simulink model "Electric_Bike"  (R2021a)
settings: Solver=VariableStepAuto  StartTime=0.0  StopTime=5  RelTol=1e-3
values from neighbouring files (symbols this model uses):
  A = [-Rm/Lm -Kb/Lm; Kt/Jeq -Beq/Jeq]    [Electric_Bicycle.m]
  AO = [A-L*C]    [Electric_Bicycle.m]
  B = [1/Lm 0;0 1/(Jeq*Em)]    [Electric_Bicycle.m]
  Beq = Bm+(B/((Em^2)*(Eg^2)))    (= 0.000601487896416)    [Electric_Bicycle.m]
  BO = [B L]    [Electric_Bicycle.m]
  C = [0 1/(Em*Eg)]    [Electric_Bicycle.m]
  CO = eye(2)    [Electric_Bicycle.m]
  DO = zeros(2,3)    [Electric_Bicycle.m]
  Eg = 0.73    [Electric_Bicycle.m]
  Em = 25    [Electric_Bicycle.m]
  Jeq = Jm+(Jb/((Em^2)*(Eg^2)))    (= 0.0135299776694)    [Electric_Bicycle.m]
  Kb = 0.16    [Electric_Bicycle.m]
  kc = place(A,B,[p1 p2])    [Electric_Bicycle.m]
  Kt = 0.16    [Electric_Bicycle.m]
  Lm = 0.003    [Electric_Bicycle.m]
  Rm = 0.85    [Electric_Bicycle.m]
settings Model: Creator=Ferna  LastModifiedBy=Ferna

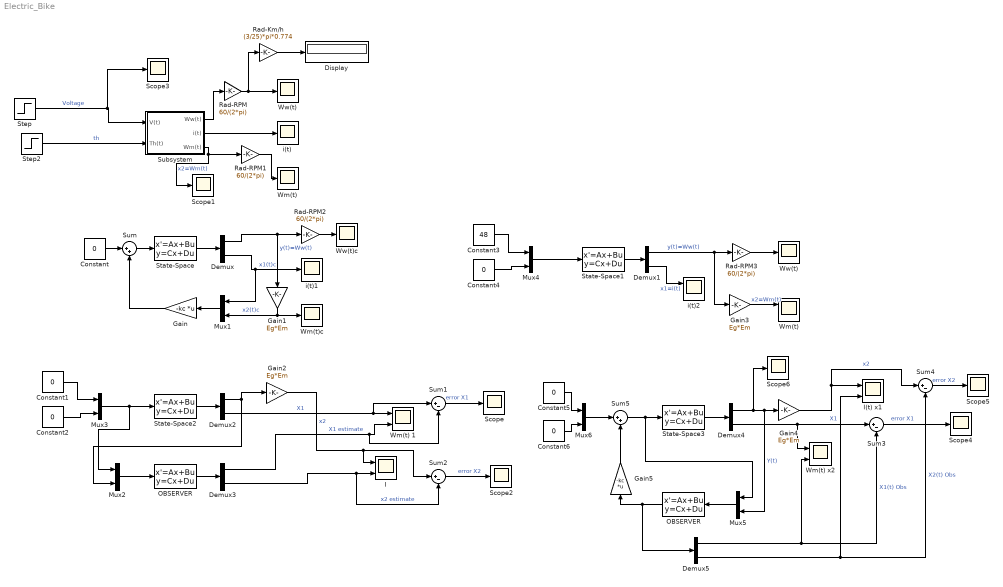
== system Electric_Bike ==
  Constant{,1..2,4..6} (6 alike) : Constant  Value=0
  Constant3 : Constant  Value=48
  Demux{,1..5} (6 alike) : Demux  Outputs=2
  Display : Display
  Gain : Gain  Gain=-kc  Multiplication=Matrix(K*u)
  Gain{1..4} (4 alike) : Gain  Gain=Eg*Em
  Gain5 : Gain  Gain=-kc  Multiplication=Matrix(K*u)
  I : Scope  NumInputPorts=2
  I(t) x1 : Scope  NumInputPorts=2
  Mux{1..6} (6 alike) : Mux  Inputs=2
  OBSERVER : StateSpace  A=AO  B=BO  C=CO  D=DO  InitialCondition=[0 100]
  "OBSERVER " : StateSpace  A=AO  B=BO  C=CO  D=DO  InitialCondition=[0 100]
  Rad-Km/h : Gain  Gain=(3/25)*pi*0.774
  Rad-RPM{,1..3} (4 alike) : Gain  Gain=60/(2*pi)
  Scope{,1..6} (7 alike) : Scope
  State-Space : StateSpace  A=A  B=B  C=[C;1 0]  D=[0 0;0 0]  InitialCondition=[0 100]
  State-Space1 : StateSpace  A=A  B=B  C=[C;1 0]  D=[0 0;0 0]  InitialCondition=[0 0]
  State-Space2 : StateSpace  A=A  B=B  C=[C;1 0]  D=[0 0;0 0]  InitialCondition=[0 100]
  State-Space3 : StateSpace  A=A  B=B  C=[C;1 0]  D=[0 0;0 0]  InitialCondition=[0 100]
  Step : Step  After=12  SampleTime=0
  Step2 : Step  After=69.3  SampleTime=0
  Subsystem : Subsystem
  Sum : Sum  Inputs=|++
  Sum{1..4} (4 alike) : Sum  Inputs=|+-
  Sum5 : Sum  Inputs=|++
  Wm(t) : Scope
  "Wm(t) " : Scope  NumInputPorts=2
  Wm(t) 1 : Scope  NumInputPorts=2
  Wm(t) x2 : Scope  NumInputPorts=2
  Wm(t)c : Scope
  Ww(t) : Scope
  "Ww(t) " : Scope
  Ww(t)c : Scope
  "i(t) " : Scope
  i(t)1 : Scope
  i(t)2 : Scope  NumInputPorts=2
  wires:
  Subsystem/2(i(t)) -> "i(t) "/1
  Subsystem/1(Ww(t)) -> Rad-RPM/1
  Subsystem/3(Wm(t)) -> Scope1/1, Rad-RPM1/1  "x2=Wm(t)"
  Rad-RPM/1 -> Rad-Km/h/1, Ww(t)/1
  Rad-RPM1/1 -> Wm(t)/1
  Rad-Km/h/1 -> Display/1
  Step/1 -> Scope3/1, Subsystem/1(V(t))  "Voltage"
  Step2/1 -> Subsystem/2(Th(t))  "th"
  State-Space/1 -> Demux/1
  Demux/2 -> Mux1/1, i(t)1/1  "x1(t)c"
  Demux/1 -> Rad-RPM2/1, Gain1/1  "y(t)=Ww(t)"
  Rad-RPM2/1 -> Ww(t)c/1
  Mux1/1 -> Gain/1
  Sum/1 -> State-Space/1
  Gain1/1 -> Mux1/2, Wm(t)c/1  "x2(t)c"
  Gain/1 -> Sum/2
  Gain3/1 -> "Wm(t) "/1  "x2=Wm(t)"
  Demux1/1 -> Rad-RPM3/1, Gain3/1  "y(t)=Ww(t)"
  Rad-RPM3/1 -> "Ww(t) "/1
  Demux1/2 -> i(t)2/1  "x1=i(t)"
  State-Space1/1 -> Demux1/1
  Constant/1 -> Sum/1
  Mux2/1 -> OBSERVER/1
  Mux3/1 -> Mux2/1, State-Space2/1
  Constant1/1 -> Mux3/1
  Constant2/1 -> Mux3/2
  Mux4/1 -> State-Space1/1
  Constant3/1 -> Mux4/1
  Constant4/1 -> Mux4/2
  State-Space2/1 -> Demux2/1
  Demux2/1 -> Gain2/1, Mux2/2
  OBSERVER/1 -> Demux3/1
  Demux3/2 -> I/2, Sum2/2  "x2 estimate"
  Demux3/1 -> Sum1/2, Wm(t) 1/2  "X1 estimate"
  Demux2/2 -> Sum1/1, Wm(t) 1/1  "X1"
  Gain2/1 -> I/1, Sum2/1  "x2"
  Sum1/1 -> Scope/1  "error X1"
  Sum2/1 -> Scope2/1  "error X2"
  Sum4/1 -> Scope5/1  "error X2"
  State-Space3/1 -> Demux4/1
  Demux4/2 -> Sum3/1, Wm(t) x2/1  "X1"
  Gain4/1 -> Sum4/1, I(t) x1/1  "x2"
  Mux5/1 -> "OBSERVER "/1
  Constant5/1 -> Mux6/1
  Demux4/1 -> Scope6/1, Mux5/2, Gain4/1  "Y(t)"
  Sum3/1 -> Scope4/1  "error X1"
  Constant6/1 -> Mux6/2
  "OBSERVER "/1 -> Demux5/1, Gain5/1
  Sum5/1 -> Mux5/1, State-Space3/1
  Gain5/1 -> Sum5/2
  Mux6/1 -> Sum5/1
  Demux5/1 -> Wm(t) x2/2, Sum3/2  "X1(t) Obs"
  Demux5/2 -> Sum4/2, I(t) x1/2  "X2(t) Obs"

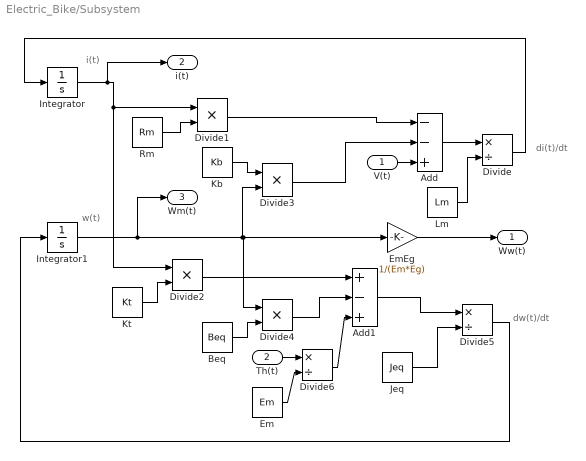
== system Electric_Bike/Subsystem ==
  note: i(t)
  note: w(t)
  note: di(t)/dt
  note: dw(t)/dt
  V(t) : Inport
  Th(t) : Inport  Port=2
  Add : Sum  Inputs=--+
  Add1 : Sum  Inputs=+-+
  Beq : Constant  Value=Beq
  Divide : Product  Inputs=*/
  Divide{1..4} (4 alike) : Product  Inputs=**
  Divide5 : Product  Inputs=*/
  Divide6 : Product  Inputs=*/
  Em : Constant  Value=Em
  EmEg : Gain  Gain=1/(Em*Eg)
  Integrator : Integrator
  Integrator1 : Integrator
  Jeq : Constant  Value=Jeq
  Kb : Constant  Value=Kb
  Kt : Constant  Value=Kt
  Lm : Constant  Value=Lm
  Rm : Constant  Value=Rm
  Ww(t) : Outport
  i(t) : Outport  Port=2
  Wm(t) : Outport  Port=3
  wires:
  Jeq/1 -> Divide5/2
  Divide4/1 -> Add1/2
  Integrator1/1 -> Wm(t)/1, EmEg/1, Divide4/1, Divide3/2
  EmEg/1 -> Ww(t)/1
  Divide2/1 -> Add1/1
  Integrator/1 -> i(t)/1, Divide2/1, Divide1/1
  Add/1 -> Divide/1
  Add1/1 -> Divide5/1
  Divide1/1 -> Add/1
  Divide5/1 -> Integrator1/1
  Lm/1 -> Divide/2
  Divide3/1 -> Add/2
  Divide/1 -> Integrator/1
  Kt/1 -> Divide2/2
  V(t)/1 -> Add/3
  Kb/1 -> Divide3/1
  Beq/1 -> Divide4/2
  Rm/1 -> Divide1/2
  Th(t)/1 -> Divide6/1
  Divide6/1 -> Add1/3
  Em/1 -> Divide6/2
